simulink model "scratchFull"  (R2020a)
settings: Solver=VariableStepAuto  StartTime=0.0  StopTime=10.0  RelTol=1e-3
undefined symbols (not defined in the file or in its folder): opt, srad
libraries: simulink x3, powerlib x1
settings Model: Creator=shrad  LastModifiedBy=shrad

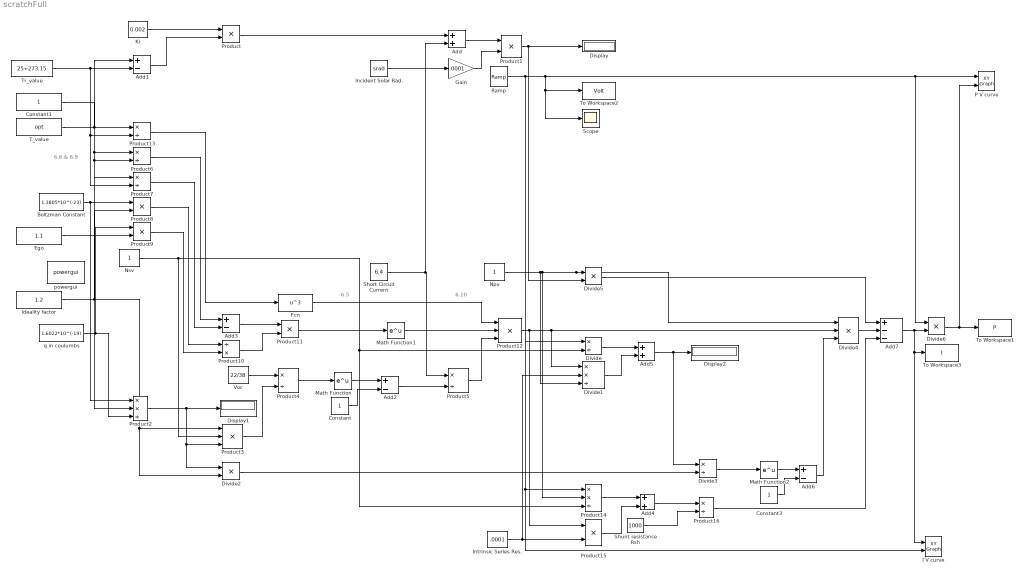
== system scratchFull ==
  note: 6.5
  note: 6.6 & 6.9
  note: 6.10
  Add : Sum
  Add{1..3,6} (4 alike) : Sum  Inputs=+-
  Add4 : Sum
  Add5 : Sum
  Add7 : Sum  Inputs=+--
  Boltzman Constant : Constant  Value=1.3805*10^(-23)
  Constant : Constant
  Constant1 : Constant
  Constant3 : Constant
  Display : Display
  Display1 : Display
  Display2 : Display
  Divide : Product  Inputs=*/
  Divide1 : Product  Inputs=**/
  Divide2 : Product
  Divide3 : Product  Inputs=*/
  Divide4 : Product  Inputs=3
  Divide5 : Product
  Divide6 : Product
  Ego : Constant  Value=1.1
  Fcn : Fcn  Expr=u^3
  Gain : Gain  Gain=.0001
  I V curve : simulink/Sinks/XY Graph  xmin=-1  xmax=22  ymin=-1  ymax=10  st=-1
  Ideality factor : Constant  Value=1.2
  Incident Solar Rad. : Constant  Value=srad
  Intrinsic Series Res. : Constant  Value=.0001
  Ki : Constant  Value=0.002
  Math Function : Math  SaturateOnIntegerOverflow=on
  Math Function1 : Math  SaturateOnIntegerOverflow=on
  Math Function2 : Math  SaturateOnIntegerOverflow=on
  Npv : Constant
  Nsv : Constant
  P V curve : simulink/Sinks/XY Graph  xmin=-1  xmax=1  ymin=-1  ymax=1  st=-1
  Product : Product
  Product1 : Product
  Product10 : Product  Inputs=/*
  Product11 : Product  Inputs=**
  Product12 : Product  Inputs=***
  Product{4..7,13,16} (6 alike) : Product  Inputs=*/
  Product14 : Product  Inputs=**/
  Product15 : Product
  Product2 : Product  Inputs=**/
  Product3 : Product  Inputs=3
  Product8 : Product  Inputs=**
  Product9 : Product  Inputs=**
  Ramp : simulink/Sources/Ramp  slope=3  start=0  InitialOutput=0
  Scope : Scope
  Short Circuit Current : Constant  Value=6.4
  Shunt resistance Rsh : Constant  Value=1000
  T_value : Constant  Value=opt
  To Workspace1 : ToWorkspace  VariableName=P  SaveFormat=Timeseries  SampleTime=-1
  To Workspace2 : ToWorkspace  VariableName=Volt  SaveFormat=Timeseries  SampleTime=-1
  To Workspace3 : ToWorkspace  VariableName=I  SaveFormat=Timeseries  SampleTime=-1
  Tr_value : Constant  Value=25+273.15
  Voc : Constant  Value=22/38
  powergui : powerlib/powergui  Priority=1  SimulationMode=Discrete  SampleTime=1e-6  frequency=60  Iterations=50  frequencyindice=0  Pbase=100e6  ErrMax=1e-4  UnitsV=kV  UnitsW=MW  buscounter=0  FunctionMessages=off  echomessages=off  EnableUseOfTLC=off  CurrentSourceSwitches=off  DisableSnubberDevices=off  DisableRonSwitches=off  DisableVfSwitches=off  DisplayEquations=off  AutomaticDiscreteSolvers=off  SolverType=Tustin  Interpol=off  ExternalGateDelay=off  methode=off  Ts=0  x0status=blocks  SPID=off  SwTol=0  HookPort=off  NonlinearTolerance=1e-4  nMaxIteration=100  ContinueOnMaxIteration=off  RestoreLinks=warning  ResistiveCurrentMeasurement=off  Frange=[0:2:500]  Ylog=off  Xlog=on  ShowGrid=off  save=off  variable=ZData  structure=0  ZoomFFT=off  StartTime=0.0  cycles=1  DisplayStyle=1  fundamental=60  FreqAxis=off  MaxFrequency=1000  frequencyindicesteady=1  RmsSteady=1  display=off
  q in coulumbs : Constant  Value=1.6022*10^(-19)
  wires:
  Math Function/1 -> Add2/1
  Gain/1 -> Product1/2
  Product3/1 -> Product4/2
  Product4/1 -> Math Function/1
  Product7/1 -> Add3/2
  Product11/1 -> Math Function1/1
  Short Circuit Current/1 -> Add/2, Product5/1
  Product10/1 -> Product11/2
  Product9/1 -> Product10/2
  Product13/1 -> Fcn/1
  Product5/1 -> Product12/3
  Npv/1 -> Divide5/1, Divide4/1, Product14/2, Divide1/3
  Product6/1 -> Add3/1
  Constant/1 -> Add2/2
  Ego/1 -> Product9/2
  Add4/1 -> Product16/1
  Shunt resistance Rsh/1 -> Product16/2
  Product14/1 -> Add4/1
  Product15/1 -> Add4/2
  Product/1 -> Add/1
  Divide/1 -> Add5/1
  Incident Solar Rad./1 -> Gain/1
  Intrinsic Series Res./1 -> Divide1/2, Product15/2
  Divide4/1 -> Add7/2
  Divide2/1 -> Divide3/2
  Divide1/1 -> Add5/2
  Product12/1 -> Divide1/1, Divide4/2, Product15/1
  Product8/1 -> Product10/1
  Add6/1 -> Divide4/3
  Math Function1/1 -> Product12/2
  Fcn/1 -> Product12/1
  Add3/1 -> Product11/1
  Divide5/1 -> Add7/1
  Product16/1 -> Add7/3
  Constant3/1 -> Add6/2
  Divide3/1 -> Math Function2/1
  Add/1 -> Product1/1
  Voc/1 -> Product4/1
  Ki/1 -> Product/1
  Add2/1 -> Product5/2
  Add1/1 -> Product/2
  Math Function2/1 -> Add6/1
  Ramp/1 -> Product14/1, I V curve/2, Scope/1, To Workspace2/1, P V curve/1, Divide6/1, Divide/1
  Nsv/1 -> Product14/3, Divide/2, Product3/2
  q in coulumbs/1 -> Product9/1, Product2/3
  Constant1/1 -> Product6/1, Product7/1
  Tr_value/1 -> Product7/2, Product13/2, Add1/2
  Divide6/1 -> P V curve/2, To Workspace1/1
  Product1/1 -> Divide5/2, Display/1
  Product2/1 -> Divide2/1, Product3/3, Display1/1
  Add7/1 -> I V curve/1, To Workspace3/1, Divide6/2
  T_value/1 -> Product2/2, Product6/2, Product13/1, Add1/1
  Add5/1 -> Display2/1, Divide3/1
  Ideality factor/1 -> Product3/1, Divide2/2, Product8/2
  Boltzman Constant/1 -> Product8/1, Product2/1
